simulink model "PubIfDecisionTOS_MDL"  (R2020b)
settings: configuration reference "DspaceConfig" (kept outside this file)
PostLoadFcn:
  | if any(exist('dsrtsu_mdlpostloadfcn', 'file') ~= 0), dsrtsu_mdlpostloadfcn('Execute', bdroot); end
InitFcn:
  | , if any(exist('dsmpb_private', 'file') ~= 0), dsmpb_private('dsmpb_mdlclblib', 'Init', bdroot); end,
undefined symbols (not defined in the file or in its folder): C_TOS_ACCEgoRAxletoFbumplength_m, C_TOS_ACCTargetFront_Flag, C_TOS_AEBJAPedObjDxThre_Val, C_TOS_AEBJAPedObjDyThre_Val, C_TOS_AEBJATargetSize_Val, C_TOS_AEBJAVehObjDxThre_Val, C_TOS_AEBJAVehObjDyThre_Val, C_TOS_AEBJuncPedTargetSize_Val, C_TOS_AEBLatObjDxThre_Val, C_TOS_AEBLatPedDyThre_Val, C_TOS_AEBLatTargetSize_Val, C_TOS_AEBLongTargetInEgoFront_Flag, C_TOS_axAbsGround_Parameter, C_TOS_CameraConfirmedFlag, C_TOS_CNsubjWidth, C_TOS_CurrentLaneCoreMinWidth_Val, C_TOS_CutInProb_Val_Zero, C_TOS_CutOutProb_Val_Zero, C_TOS_D2R_Val, C_TOS_DefaultValueObjectToCenterLine_dy, C_TOS_EgoCarWidth_Val, C_TOS_EgoDxRefPoint_m, C_TOS_EgoRAxletoFbumplength_m, C_TOS_HalfWidthVehicle_Con, C_TOS_HWA_CurrentLaneFlag, C_TOS_HWA_LeftLaneFlag, C_TOS_HWA_MovingDir_Vaild, C_TOS_HWA_MovState_Vaild, C_TOS_HWA_RightLaneFlag, C_TOS_LaneLineCourseErrorFront, C_TOS_LaneLineCourseErrorRear, C_TOS_MotorbikeDefaultWidth_m, C_TOS_NumberOfEffectiveTargets, C_TOS_Obj_Age_Val, C_TOS_Objdx_Constraint_Val, C_TOS_ObjectDefaultWidth_m, C_TOS_ObjInCurrentLane_Val, C_TOS_ObjInCurrentLaneValid, C_TOS_ObjInLeftLaneValid, C_TOS_ObjInRightLaneValid, C_TOS_ObjNotInCurrentLane_Val, C_TOS_ObjNotREElementType, C_TOS_ObjPredictDis_dy_ConstantVal_Zeros, C_TOS_ObjToCenterLine_ConstantVal_Zeros, C_TOS_OFMObjIDInvilad_Val, C_TOS_PIL_LatDisCons_Val_zero, C_TOS_PIL_ObjectCutInFlag_b, C_TOS_PIL_ObjectCutOutFlag_b, C_TOS_PIL_ObjLaneProb_al_Val, C_TOS_PP_ObjFusType_FC_Confirm_b, C_TOS_PP_ObjFusType_FC_FR_Confirm_b, C_TOS_PP_ObjFusType_FR_Confirm_b, C_TOS_RE_80BoolDefault_Val, C_TOS_RE_80Single181Default_Val, C_TOS_RE_80Single255Default_Val, C_TOS_RE_80Uint8Default_Val, C_TOS_RE_D2R, C_TOS_RE_D_180_Val, C_TOS_RE_InvalidObjectID_Val, C_TOS_RE_InvalidTargetChainDir_Val ... (+142)
libraries: simulink x1650, TOS_LIB x361, canfdmsglib x14
(part 31 of 69)

== system PubIfDecisionTOS_MDL/TOS_20201112/TOS_2012080320/TOS/LC_LCKie_ELK/TOS_HWA/RightLane/HWA_Object_PreConfirm/HWA_Object_PreConfirm ==
  PP_ObjFusType_FC_FR_Confirm : Inport  Partition=on  PartitionDimension=1  PartitionWidth=1  PartitionOffset=0
  PP_ObjFusType_FR_Confirm : Inport  Port=2  Partition=on  PartitionDimension=1  PartitionWidth=1  PartitionOffset=0
  PP_ObjFusType_FC_Confirm : Inport  Port=3  Partition=on  PartitionDimension=1  PartitionWidth=1  PartitionOffset=0
  Object_ID : Inport  Port=4  OutDataTypeStr=uint8  Partition=on  PartitionDimension=1  PartitionWidth=1  PartitionOffset=0
  Obj_MovingState : Inport  Port=5  Partition=on  PartitionDimension=1  PartitionWidth=1  PartitionOffset=0
  Obj_Dx : Inport  Port=6  Partition=on  PartitionDimension=1  PartitionWidth=1  PartitionOffset=0
  Object_ObstacleProb : Inport  Port=7  Partition=on  PartitionDimension=1  PartitionWidth=1  PartitionOffset=0
  Object_DY : Inport  Port=8  Partition=on  PartitionDimension=1  PartitionWidth=1  PartitionOffset=0
  Object_ObjType : Inport  Port=9  Partition=on  PartitionDimension=1  PartitionWidth=1  PartitionOffset=0
  Compare To Constant : simulink/Logic and Bit Operations/Compare To Constant  relop=~=  const=C_TOS_OFMObjIDInvilad_Val  OutDataTypeStr=boolean
      settings: AttributesFormatString=C_TOS_OFMObjIDInvilad_Val = 0
  Compare To Constant1 : simulink/Logic and Bit Operations/Compare To Constant  relop=>=  const=single(7)  OutDataTypeStr=boolean
      settings: AttributesFormatString=dx >= single(0)
  Compare To Constant2 : simulink/Logic and Bit Operations/Compare To Constant  relop=<  const=single(7)  OutDataTypeStr=boolean
      settings: AttributesFormatString=dx >= single(0)
  Default : Subsystem  TreatAsAtomicUnit=on
  For Each : ForEach  DisableCoverage=on
  HWA_Object_PreConfirm : Subsystem
  HWA_Object_PreConfirmDefault1 : Subsystem  TreatAsAtomicUnit=on
  If1 : If  NumInputs=2  IfExpression=u1 == 1  ElseIfExpressions=u2 == 1
  Logical Operator1 : Logic  AllPortsSameDT=off  OutDataTypeStr=boolean
  Logical Operator3 : Logic  AllPortsSameDT=off  OutDataTypeStr=boolean
  Merge{,1,3..5} (5 alike) : Merge  Inputs=3
  TOS_HWA_TargetPre_Confirm_Filt_Flag : Outport  ConcatenationDimension=1
  TOS_HWA_TargetPre_FusionTypeFlag_ObserVale : Outport  Port=2  ConcatenationDimension=1
  TOS_HWA_TargetPre_PassedbyTarget_ObserVale : Outport  Port=3  ConcatenationDimension=1
  TOS_HWA_TargetPre_ObjType_ObserVale : Outport  Port=4  ConcatenationDimension=1
  TOS_HWA_DyConfirm_ObserVale : Outport  Port=5  ConcatenationDimension=1
  wires:
  PP_ObjFusType_FC_FR_Confirm/1 -> HWA_Object_PreConfirm/2(PP_ObjFusType_FC_FR_Confirm)
  PP_ObjFusType_FR_Confirm/1 -> HWA_Object_PreConfirm/3(PP_ObjFusType_FR_Confirm)
  Compare To Constant/1 -> Logical Operator1/1, Logical Operator3/1
  Object_ID/1 -> [Object_ID], Compare To Constant/1
  If1/3 -> Default/Action
  If1/1 -> HWA_Object_PreConfirm/Action
  PP_ObjFusType_FC_Confirm/1 -> HWA_Object_PreConfirm/4(PP_ObjFusType_FC_Confirm)
  Obj_MovingState/1 -> HWA_Object_PreConfirm/5(Obj_MovingState)
  Obj_Dx/1 -> HWA_Object_PreConfirm/6(Obj_Dx)
  Object_ObstacleProb/1 -> HWA_Object_PreConfirm/7(Object_ObstacleProb)
  Object_DY/1 -> HWA_Object_PreConfirm/8(Object_DY)
  [Object_ID] -> HWA_Object_PreConfirm/1(Object_ID)
  Object_ObjType/1 -> HWA_Object_PreConfirm/9(Object_ObjType)
  HWA_Object_PreConfirm/1(TOS_HWA_TargetPre_Confirm_Filt_Flag) -> Merge/2
  HWA_Object_PreConfirm/2(TOS_HWA_TargetPre_FusionTypeFlag_ObserVale) -> Merge5/2
  HWA_Object_PreConfirm/3(TOS_HWA_TargetPre_PassedbyTarget_Flag_ObserVale) -> Merge1/2
  HWA_Object_PreConfirm/4(TOS_HWA_TargetPre_ObjType_ObserVale) -> Merge3/2
  HWA_Object_PreConfirm/5(TOS_HWA_DyConfirm_ObserVale) -> Merge4/2
  Merge/1 -> TOS_HWA_TargetPre_Confirm_Filt_Flag/1
  Merge5/1 -> TOS_HWA_TargetPre_FusionTypeFlag_ObserVale/1
  Merge1/1 -> TOS_HWA_TargetPre_PassedbyTarget_ObserVale/1
  Merge3/1 -> TOS_HWA_TargetPre_ObjType_ObserVale/1
  Merge4/1 -> TOS_HWA_DyConfirm_ObserVale/1
  [Obj_Dx] -> Compare To Constant1/1, Compare To Constant2/1
  Compare To Constant1/1 -> Logical Operator3/2
  Compare To Constant2/1 -> Logical Operator1/2
  Logical Operator3/1 -> If1/1
  Logical Operator1/1 -> If1/2
  If1/2 -> HWA_Object_PreConfirmDefault1/Action
  HWA_Object_PreConfirmDefault1/1(TOS_HWA_TargetPre_Confirm_Filt_Flag) -> Merge/1
  HWA_Object_PreConfirmDefault1/2(TOS_HWA_TargetPre_FusionTypeFlag_ObserVale) -> Merge5/1
  HWA_Object_PreConfirmDefault1/3(TOS_HWA_TargetPre_PassedbyTarget_Flag_ObserVale) -> Merge1/1
  HWA_Object_PreConfirmDefault1/4(TOS_HWA_TargetPre_ObjType_ObserVale) -> Merge3/1
  HWA_Object_PreConfirmDefault1/5(TOS_HWA_DyConfirm_ObserVale) -> Merge4/1
  Default/5(TOS_HWA_DyConfirm_ObserVale) -> Merge4/3
  Default/4(TOS_HWA_TargetPre_ObjType_ObserVale) -> Merge3/3
  Default/3(TOS_HWA_TargetPre_PassedbyTarget_Flag_ObserVale) -> Merge1/3
  Default/2(TOS_HWA_TargetPre_FusionTypeFlag_ObserVale) -> Merge5/3
  Default/1(TOS_HWA_TargetPre_Confirm_Filt_Flag) -> Merge/3

== system PubIfDecisionTOS_MDL/TOS_20201112/TOS_2012080320/TOS/LC_LCKie_ELK/TOS_HWA/RightLane/TOS_HWA_RightLane/TOS_HWA_RightLane ==
  HWA_RightLane_ObjIndex : Inport  Partition=on  PartitionDimension=1  PartitionWidth=1  PartitionOffset=0
  PP_ObjMovingDirSignalProcessing : Inport  Port=2
  Object_VX : Inport  Port=3
  Object_VY : Inport  Port=4
  Object_Type : Inport  Port=5
  Object_MovingState : Inport  Port=6
  TOS_TLJ_RightLaneConfirm_Flag : Inport  Port=7
  Object_DX : Inport  Port=8
  Object_DY : Inport  Port=9
  Object_Fus_Type : Inport  Port=10
  Object_HeadingAngle : Inport  Port=11
  PP_ObjFusType_FC_FR_Confirm : Inport  Port=12
  PP_ObjFusType_FR_Confirm : Inport  Port=13
  PP_ObjFusType_FC_Confirm : Inport  Port=14
  VIE_EgoVelocity : Inport  Port=15
  Compare To Constant : simulink/Logic and Bit Operations/Compare To Constant  relop===  const=C_TOS_OFMObjIDInvilad_Val  OutDataTypeStr=boolean
      settings: AttributesFormatString=C_TOS_OFMObjIDInvilad_Val = 0
  Constant : Constant  Value=0  OutDataTypeStr=uint8
  Constant1 : Constant  Value=0  OutDataTypeStr=uint8
  Constant2 : Constant  Value=0  OutDataTypeStr=uint8
  Constant4 : Constant  Value=C_TOS_ObjInRightLaneValid  OutDataTypeStr=uint8
      settings: AttributesFormatString=C_TOS_ObjInRightLaneValid = 3
  For Each : ForEach  DisableCoverage=on
  If : If  IfExpression=u1 ~= 0
  Merge{1..11} (11 alike) : Merge
  Switch : Switch  Criteria=u2 ~= 0
  Switch1 : Switch  Criteria=u2 ~= 0
  Switch2 : Switch  Criteria=u2 ~= 0
  TOS_HWA : Subsystem
  TOS_HWA_Default : Subsystem  TreatAsAtomicUnit=on
  TOS_HWA_TargetInRightLane_b : Outport  ConcatenationDimension=1
  TOS_HWA_RightFront_TargConfirm_b : Outport  Port=2  ConcatenationDimension=1
  TOS_HWA_RightRear_TargConfirm_b : Outport  Port=3  ConcatenationDimension=1
  TOS_HWA_RightFront_FusType_ObserVale : Outport  Port=4  ConcatenationDimension=1
  TOS_HWA_InRightLane_Front_Flag_ObserVale : Outport  Port=5  ConcatenationDimension=1
  TOS_HWA_RightFront_TargMovDir_ObserVale : Outport  Port=6  ConcatenationDimension=1
  TOS_HWA_RightRear_MovState_ObserVale : Outport  Port=7  ConcatenationDimension=1
  TOS_HWA_RightRear_FusionType_ObserVale : Outport  Port=8  ConcatenationDimension=1
  TOS_HWA_InRightLane_Rear_Flag_ObserVale : Outport  Port=9  ConcatenationDimension=1
  TOS_HWA_RightRear_TargetMovingDir_ObserVale : Outport  Port=10  ConcatenationDimension=1
  TOS_HWA_RightRear_DyConfirm_ObserVale : Outport  Port=11  ConcatenationDimension=1
  wires:
  If/1 -> TOS_HWA_Default/Action
  Compare To Constant/1 -> If/1
  If/2 -> TOS_HWA/Action
  PP_ObjMovingDirSignalProcessing/1 -> TOS_HWA/2(PP_ObjMovingDirSignalProcessing)
  Object_VX/1 -> TOS_HWA/3(Object_VX)
  Object_VY/1 -> TOS_HWA/4(Object_VY)
  Object_Type/1 -> TOS_HWA/5(Object_Type)
  Object_MovingState/1 -> TOS_HWA/6(object_MovingState)
  TOS_TLJ_RightLaneConfirm_Flag/1 -> TOS_HWA/7(TOS_TLJ_RightLaneConfirm_Flag)
  Object_DX/1 -> TOS_HWA/8(Object_DX)  "Object_DX"
  Object_Fus_Type/1 -> TOS_HWA/10(Object_Fus_Type)
  Object_HeadingAngle/1 -> TOS_HWA/11(Object_HeadingAngle)  "Object_HeadingAngle"
  HWA_RightLane_ObjIndex/1 -> [HWA_RightLane_ObjIndex], Compare To Constant/1
  [HWA_RightLane_ObjIndex] -> Switch/1
  Constant/1 -> Switch/3
  Switch/1 -> TOS_HWA_RightFront_TargConfirm_b/1
  Switch1/1 -> TOS_HWA_RightRear_TargConfirm_b/1
  Constant1/1 -> Switch1/3
  [HWA_RightLane_ObjIndex] -> Switch1/1
  [HWA_RightLane_ObjIndex] -> TOS_HWA/1(HWA_RightLane_ObjIndex)
  Constant4/1 -> Switch2/1
  Constant2/1 -> Switch2/3
  Switch2/1 -> TOS_HWA_TargetInRightLane_b/1
  PP_ObjFusType_FC_Confirm/1 -> TOS_HWA/14(PP_ObjFusType_FC_Confirm)
  PP_ObjFusType_FC_FR_Confirm/1 -> TOS_HWA/12(PP_ObjFusType_FC_FR_Confirm)
  PP_ObjFusType_FR_Confirm/1 -> TOS_HWA/13(PP_ObjFusType_FR_Confirm)
  VIE_EgoVelocity/1 -> TOS_HWA/15(VIE_EgoVelocity)
  TOS_HWA/11(TOS_HWA_RightRear_DyConfirm_ObserVale) -> Merge11/2
  TOS_HWA/1(TOS_HWA_TargetInRightLane_b) -> Merge3/2
  TOS_HWA/2(TOS_HWA_RightFront_TargConfirm_b) -> Merge4/2
  TOS_HWA/3(TOS_HWA_RightRear_TargConfirm_b) -> Merge5/2
  TOS_HWA/4(TOS_HWA_RightFront_FusType_ObserVale) -> Merge1/2
  TOS_HWA/5(TOS_HWA_InRightLane_Front_Flag_ObserVale) -> Merge2/2
  TOS_HWA/6(TOS_HWA_RightFront_TargMovDir_ObserVale) -> Merge6/2
  TOS_HWA/7(TOS_HWA_RightRear_MovState_ObserVale) -> Merge7/2
  TOS_HWA/8(TOS_HWA_RightRear_FusionType_ObserVale) -> Merge8/2
  TOS_HWA/9(TOS_HWA_InRightLane_Rear_Flag_ObserVale) -> Merge9/2
  TOS_HWA/10(TOS_HWA_RightRear_TargetMovingDir_ObserVale) -> Merge10/2
  TOS_HWA_Default/1(TOS_HWA_TargetInRightLane_b) -> Merge3/1
  Merge4/1 -> Switch/2
  Merge5/1 -> Switch1/2
  TOS_HWA_Default/2(TOS_HWA_RightFront_TargConfirm_b) -> Merge4/1
  TOS_HWA_Default/3(TOS_HWA_RightRear_TargConfirm_b) -> Merge5/1
  Merge3/1 -> Switch2/2
  Merge1/1 -> TOS_HWA_RightFront_FusType_ObserVale/1
  Merge11/1 -> TOS_HWA_RightRear_DyConfirm_ObserVale/1
  Merge2/1 -> TOS_HWA_InRightLane_Front_Flag_ObserVale/1
  Merge6/1 -> TOS_HWA_RightFront_TargMovDir_ObserVale/1
  Merge7/1 -> TOS_HWA_RightRear_MovState_ObserVale/1
  Merge8/1 -> TOS_HWA_RightRear_FusionType_ObserVale/1
  Merge9/1 -> TOS_HWA_InRightLane_Rear_Flag_ObserVale/1
  Merge10/1 -> TOS_HWA_RightRear_TargetMovingDir_ObserVale/1
  TOS_HWA_Default/4(TOS_HWA_RightFront_FusType_ObserVale) -> Merge1/1
  TOS_HWA_Default/5(TOS_HWA_InRightLane_Front_Flag_ObserVale) -> Merge2/1
  TOS_HWA_Default/6(TOS_HWA_RightFront_TargMovDir_ObserVale) -> Merge6/1
  TOS_HWA_Default/7(TOS_HWA_RightRear_MovState_ObserVale) -> Merge7/1
  TOS_HWA_Default/8(TOS_HWA_RightRear_FusionType_ObserVale) -> Merge8/1
  TOS_HWA_Default/9(TOS_HWA_InRightLane_Rear_Flag_ObserVale) -> Merge9/1
  TOS_HWA_Default/10(TOS_HWA_RightRear_TargetMovingDir_ObserVale) -> Merge10/1
  TOS_HWA_Default/11(TOS_HWA_RightRear_DyConfirm_ObserVale) -> Merge11/1
  Object_DY/1 -> TOS_HWA/9(Object_DY)  "Object_DY"

== system PubIfDecisionTOS_MDL/TOS_20201112/TOS_2012080320/TOS/P0_Trajectory_V1.0/CordinatConvert/CordinatConvert/CordinatConvert/TrackRecord_CordinatConvert ==
  note: 清除后方 -20m以后目标（不清除，历史点一直存在对下一次拟合有影响）
  note: 默认数组，无目标时，不坐标转换
  EgoVeh_OffsetX : Inport
  EgoVeh_OffsetY : Inport  Port=2
  EgoVeh_OffsetAngle : Inport  Port=3
  P0_dx_TrackRecord_K1 : Inport  Port=4  Partition=on  PartitionDimension=1  PartitionWidth=1  PartitionOffset=0
  P0_dy_TrackRecord_K1 : Inport  Port=5  Partition=on  PartitionDimension=1  PartitionWidth=1  PartitionOffset=0
  P0_Counter_TrackRecord : Inport  Port=6  Partition=on  PartitionDimension=1  PartitionWidth=1  PartitionOffset=0
  P0_ID_TrackRecord_K1 : Inport  Port=7  Partition=on  PartitionDimension=1  PartitionWidth=1  PartitionOffset=0
  Bus Creator : BusCreator  Inputs=7
  Bus Selector : BusSelector  OutputSignals=P0_dx_TrackRecord_K1,P0_dy_TrackRecord_K1,P0_Counter_TrackRecord
  Bus Selector1 : BusSelector  OutputSignals=EgoVeh_OffsetX,EgoVeh_OffsetY,EgoVeh_OffsetAngle,P0_dx_TrackRecord_K1,P0_dy_TrackRecord_K1,P0_Counter_TrackRecord,P0_ID_TrackRecord_K1
  Bus Selector2 : BusSelector  OutputSignals=P0_dx_TrackRecord_K1
  Compare To Constant : simulink/Logic and Bit Operations/Compare To Constant  relop===  const=single(0)  OutDataTypeStr=boolean
      settings: AttributesFormatString=Invilad_Val = single(0)
  Compare To Constant1 : simulink/Logic and Bit Operations/Compare To Constant  relop===  const=single(0)  OutDataTypeStr=boolean
      settings: AttributesFormatString=Invilad_Val = single(0)
  Compare To Constant2 : simulink/Logic and Bit Operations/Compare To Constant  relop===  const=uint32(0)  OutDataTypeStr=boolean
      settings: AttributesFormatString=Invilad_Val = uint32(0)
  Compare To Constant3 : simulink/Logic and Bit Operations/Compare To Constant  relop=<=  const=single(-20)  OutDataTypeStr=boolean
      settings: AttributesFormatString=single(-20)
  CordinatConvertDefault : Subsystem  TreatAsAtomicUnit=on
  For Each : ForEach  DisableCoverage=on
  If : If  IfExpression=u1 == 1
  Logical Operator1 : Logic  Inputs=3  AllPortsSameDT=off  OutDataTypeStr=boolean
  Logical Operator2 : Logic  Operator=OR  AllPortsSameDT=off  OutDataTypeStr=boolean
  Merge{1..4} (4 alike) : Merge
  TrackRecord_CordinatConvert : Subsystem
  P0_dx_TrackRecord_CordinatConvert_K1 : Outport  ConcatenationDimension=1
  P0_dy_TrackRecord_CordinatConvert_K1 : Outport  Port=2  ConcatenationDimension=1
  P0_Counter_TrackRecord_CordinatConvert_K1 : Outport  Port=3  ConcatenationDimension=1
  P0_ID_TrackRecord_CordinatConvert_K1 : Outport  Port=4  ConcatenationDimension=1
  wires:
  Merge3/1 -> P0_Counter_TrackRecord_CordinatConvert_K1/1
  Merge1/1 -> P0_dy_TrackRecord_CordinatConvert_K1/1
  Merge2/1 -> P0_dx_TrackRecord_CordinatConvert_K1/1
  CordinatConvertDefault/3(P0_Counter_TrackRecord_CordinatConvert_K1) -> Merge3/1
  CordinatConvertDefault/2(P0_dy_TrackRecord_CordinatConvert_K1) -> Merge1/1
  CordinatConvertDefault/1(P0_dx_TrackRecord_CordinatConvert_K1) -> Merge2/1
  TrackRecord_CordinatConvert/3(P0_Counter_TrackRecord_CordinatConvert_K1) -> Merge3/2
  TrackRecord_CordinatConvert/2(P0_dy_TrackRecord_CordinatConvert_K1) -> Merge1/2
  TrackRecord_CordinatConvert/1(P0_dx_TrackRecord_CordinatConvert_K1) -> Merge2/2
  Bus Selector1/6 -> TrackRecord_CordinatConvert/6(P0_Counter_TrackRecord)  "<P0_Counter_TrackRecord>"
  Bus Selector1/5 -> TrackRecord_CordinatConvert/5(P0_dy_TrackRecord_K1)  "<P0_dy_TrackRecord_K1>"
  Bus Selector1/4 -> TrackRecord_CordinatConvert/4(P0_dx_TrackRecord_K1)  "<P0_dx_TrackRecord_K1>"
  Bus Selector1/3 -> TrackRecord_CordinatConvert/3(EgoVeh_OffsetAngle)  "<EgoVeh_OffsetAngle>"
  Bus Selector1/2 -> TrackRecord_CordinatConvert/2(EgoVeh_OffsetY)  "<EgoVeh_OffsetY>"
  Bus Selector1/1 -> TrackRecord_CordinatConvert/1(EgoVeh_OffsetX)  "<EgoVeh_OffsetX>"
  [TrackRecord_CordinatConvert] -> Bus Selector1/1
  If/2 -> TrackRecord_CordinatConvert/Action
  If/1 -> CordinatConvertDefault/Action
  Logical Operator2/1 -> If/1
  Compare To Constant2/1 -> Logical Operator1/3
  Compare To Constant1/1 -> Logical Operator1/2
  Compare To Constant/1 -> Logical Operator1/1
  Bus Selector/3 -> Compare To Constant2/1  "<P0_Counter_TrackRecord>"
  Bus Selector/2 -> Compare To Constant1/1  "<P0_dy_TrackRecord_K1>"
  Bus Selector/1 -> Compare To Constant/1  "<P0_dx_TrackRecord_K1>"
  Bus Creator/1 -> Bus Selector2/1, Bus Selector/1, [TrackRecord_CordinatConvert]
  EgoVeh_OffsetY/1 -> Bus Creator/2  "EgoVeh_OffsetY"
  EgoVeh_OffsetAngle/1 -> Bus Creator/3  "EgoVeh_OffsetAngle"
  P0_Counter_TrackRecord/1 -> Bus Creator/6  "P0_Counter_TrackRecord"
  P0_dy_TrackRecord_K1/1 -> Bus Creator/5  "P0_dy_TrackRecord_K1"
  EgoVeh_OffsetX/1 -> Bus Creator/1  "EgoVeh_OffsetX"
  P0_dx_TrackRecord_K1/1 -> Bus Creator/4  "P0_dx_TrackRecord_K1"
  P0_ID_TrackRecord_K1/1 -> Bus Creator/7  "P0_ID_TrackRecord_K1"
  Bus Selector1/7 -> TrackRecord_CordinatConvert/7(P0_ID_TrackRecord_K1)  "<P0_ID_TrackRecord_K1>"
  Merge4/1 -> P0_ID_TrackRecord_CordinatConvert_K1/1
  TrackRecord_CordinatConvert/4(P0_ID_TrackRecord_CordinatConvert_K2) -> Merge4/2
  CordinatConvertDefault/4(P0_ID_TrackRecord_CordinatConvert_K1) -> Merge4/1
  Bus Selector2/1 -> Compare To Constant3/1  "<P0_dx_TrackRecord_K1>"
  Compare To Constant3/1 -> Logical Operator2/2
  Logical Operator1/1 -> Logical Operator2/1

== system PubIfDecisionTOS_MDL/TOS_20201112/TOS_2012080320/TOS/P0_Trajectory_V1.0/CordinatConvert/CordinatConvert1/CordinatConvert/TrackRecord_CordinatConvert ==
  note: 默认数组，无目标时，不坐标转换
  note: 清除后方 -20m以后目标（不清除，历史点一直存在对下一次拟合有影响）
  EgoVeh_OffsetX : Inport
  EgoVeh_OffsetY : Inport  Port=2
  EgoVeh_OffsetAngle : Inport  Port=3
  P0_dx_TrackRecord_K1 : Inport  Port=4  Partition=on  PartitionDimension=1  PartitionWidth=1  PartitionOffset=0
  P0_dy_TrackRecord_K1 : Inport  Port=5  Partition=on  PartitionDimension=1  PartitionWidth=1  PartitionOffset=0
  P0_Counter_TrackRecord : Inport  Port=6  Partition=on  PartitionDimension=1  PartitionWidth=1  PartitionOffset=0
  P0_ID_TrackRecord_K1 : Inport  Port=7  Partition=on  PartitionDimension=1  PartitionWidth=1  PartitionOffset=0
  Bus Creator : BusCreator  Inputs=7
  Bus Selector : BusSelector  OutputSignals=P0_dx_TrackRecord_K1,P0_dy_TrackRecord_K1,P0_Counter_TrackRecord
  Bus Selector1 : BusSelector  OutputSignals=EgoVeh_OffsetX,EgoVeh_OffsetY,EgoVeh_OffsetAngle,P0_dx_TrackRecord_K1,P0_dy_TrackRecord_K1,P0_Counter_TrackRecord,P0_ID_TrackRecord_K1
  Bus Selector2 : BusSelector  OutputSignals=P0_dx_TrackRecord_K1
  Compare To Constant : simulink/Logic and Bit Operations/Compare To Constant  relop===  const=single(0)  OutDataTypeStr=boolean
      settings: AttributesFormatString=Invilad_Val = single(0)
  Compare To Constant1 : simulink/Logic and Bit Operations/Compare To Constant  relop===  const=single(0)  OutDataTypeStr=boolean
      settings: AttributesFormatString=Invilad_Val = single(0)
  Compare To Constant2 : simulink/Logic and Bit Operations/Compare To Constant  relop===  const=uint32(0)  OutDataTypeStr=boolean
      settings: AttributesFormatString=Invilad_Val = uint32(0)
  Compare To Constant3 : simulink/Logic and Bit Operations/Compare To Constant  relop=<=  const=single(-20)  OutDataTypeStr=boolean
      settings: AttributesFormatString=single(-20)
  CordinatConvertDefault : Subsystem  TreatAsAtomicUnit=on
  For Each : ForEach  DisableCoverage=on
  If : If  IfExpression=u1 == 1
  Logical Operator1 : Logic  Inputs=3  AllPortsSameDT=off  OutDataTypeStr=boolean
  Logical Operator2 : Logic  Operator=OR  AllPortsSameDT=off  OutDataTypeStr=boolean
  Merge{1..4} (4 alike) : Merge
  TrackRecord_CordinatConvert : Subsystem
  P0_dx_TrackRecord_CordinatConvert_K1 : Outport  ConcatenationDimension=1
  P0_dy_TrackRecord_CordinatConvert_K1 : Outport  Port=2  ConcatenationDimension=1
  P0_Counter_TrackRecord_CordinatConvert_K1 : Outport  Port=3  ConcatenationDimension=1
  P0_ID_TrackRecord_CordinatConvert_K1 : Outport  Port=4  ConcatenationDimension=1
  wires:
  Logical Operator1/1 -> Logical Operator2/1
  Compare To Constant3/1 -> Logical Operator2/2
  Bus Selector2/1 -> Compare To Constant3/1  "<P0_dx_TrackRecord_K1>"
  CordinatConvertDefault/4(P0_ID_TrackRecord_CordinatConvert_K1) -> Merge4/1
  TrackRecord_CordinatConvert/4(P0_ID_TrackRecord_CordinatConvert_K2) -> Merge4/2
  Merge4/1 -> P0_ID_TrackRecord_CordinatConvert_K1/1
  Bus Selector1/7 -> TrackRecord_CordinatConvert/7(P0_ID_TrackRecord_K1)  "<P0_ID_TrackRecord_K1>"
  P0_ID_TrackRecord_K1/1 -> Bus Creator/7  "P0_ID_TrackRecord_K1"
  P0_dx_TrackRecord_K1/1 -> Bus Creator/4  "P0_dx_TrackRecord_K1"
  EgoVeh_OffsetX/1 -> Bus Creator/1  "EgoVeh_OffsetX"
  P0_dy_TrackRecord_K1/1 -> Bus Creator/5  "P0_dy_TrackRecord_K1"
  P0_Counter_TrackRecord/1 -> Bus Creator/6  "P0_Counter_TrackRecord"
  EgoVeh_OffsetAngle/1 -> Bus Creator/3  "EgoVeh_OffsetAngle"
  EgoVeh_OffsetY/1 -> Bus Creator/2  "EgoVeh_OffsetY"
  Bus Creator/1 -> [TrackRecord_CordinatConvert], Bus Selector/1, Bus Selector2/1
  Bus Selector/1 -> Compare To Constant/1  "<P0_dx_TrackRecord_K1>"
  Bus Selector/2 -> Compare To Constant1/1  "<P0_dy_TrackRecord_K1>"
  Bus Selector/3 -> Compare To Constant2/1  "<P0_Counter_TrackRecord>"
  Compare To Constant/1 -> Logical Operator1/1
  Compare To Constant1/1 -> Logical Operator1/2
  Compare To Constant2/1 -> Logical Operator1/3
  Logical Operator2/1 -> If/1
  If/1 -> CordinatConvertDefault/Action
  If/2 -> TrackRecord_CordinatConvert/Action
  [TrackRecord_CordinatConvert] -> Bus Selector1/1
  Bus Selector1/1 -> TrackRecord_CordinatConvert/1(EgoVeh_OffsetX)  "<EgoVeh_OffsetX>"
  Bus Selector1/2 -> TrackRecord_CordinatConvert/2(EgoVeh_OffsetY)  "<EgoVeh_OffsetY>"
  Bus Selector1/3 -> TrackRecord_CordinatConvert/3(EgoVeh_OffsetAngle)  "<EgoVeh_OffsetAngle>"
  Bus Selector1/4 -> TrackRecord_CordinatConvert/4(P0_dx_TrackRecord_K1)  "<P0_dx_TrackRecord_K1>"
  Bus Selector1/5 -> TrackRecord_CordinatConvert/5(P0_dy_TrackRecord_K1)  "<P0_dy_TrackRecord_K1>"
  Bus Selector1/6 -> TrackRecord_CordinatConvert/6(P0_Counter_TrackRecord)  "<P0_Counter_TrackRecord>"
  TrackRecord_CordinatConvert/1(P0_dx_TrackRecord_CordinatConvert_K1) -> Merge2/2
  TrackRecord_CordinatConvert/2(P0_dy_TrackRecord_CordinatConvert_K1) -> Merge1/2
  TrackRecord_CordinatConvert/3(P0_Counter_TrackRecord_CordinatConvert_K1) -> Merge3/2
  CordinatConvertDefault/1(P0_dx_TrackRecord_CordinatConvert_K1) -> Merge2/1
  CordinatConvertDefault/2(P0_dy_TrackRecord_CordinatConvert_K1) -> Merge1/1
  CordinatConvertDefault/3(P0_Counter_TrackRecord_CordinatConvert_K1) -> Merge3/1
  Merge2/1 -> P0_dx_TrackRecord_CordinatConvert_K1/1
  Merge1/1 -> P0_dy_TrackRecord_CordinatConvert_K1/1
  Merge3/1 -> P0_Counter_TrackRecord_CordinatConvert_K1/1

== system PubIfDecisionTOS_MDL/TOS_20201112/TOS_2012080320/TOS/P0_Trajectory_V1.0/TrackRecord/Subsystem1/P0_Position_Num/EndPosition ==
  P0_dx_TrackRecord_CordinatConvert_K1 : Inport
  P0_dy_TrackRecord_CordinatConvert_K1 : Inport  Port=2
  P0_ObjVaild_TrackRecord_CordinatConvert_K1 : Inport  Port=3
  P0_Trajectory_TrackRecord_Num : Inport  Port=4
  Abs : Abs
  Abs1 : Abs
  Abs2 : Abs
  Add : Sum  OutDataTypeStr=int32
  Compare To Constant1 : simulink/Logic and Bit Operations/Compare To Constant  relop=~=  const=single(0)  OutDataTypeStr=boolean
      settings: AttributesFormatString=single(0)
  Compare To Constant10 : simulink/Logic and Bit Operations/Compare To Constant  relop===  const=uint32(0)  OutDataTypeStr=boolean
      settings: AttributesFormatString=uint32(0)
  Compare To Constant2 : simulink/Logic and Bit Operations/Compare To Constant  relop=~=  const=uint32(0)  OutDataTypeStr=boolean
      settings: AttributesFormatString=uint32(0)
  Compare To Constant5 : simulink/Logic and Bit Operations/Compare To Constant  relop=~=  const=single(0)  OutDataTypeStr=boolean
      settings: AttributesFormatString=single(0)
  Constant : Constant  OutDataTypeStr=int32
  Data Type Conversion : DataTypeConversion  OutDataTypeStr=uint32
  Index Vector{,1..5} (6 alike) : MultiPortSwitch  Inputs=1
  Logical Operator2 : Logic  Inputs=4  AllPortsSameDT=off  OutDataTypeStr=boolean
  P0_dx_TrackRecord_CordinatConvert_K2 : InportShadow
  P0_dy_TrackRecord_CordinatConvert_K2 : InportShadow  Port=2
  Saturation : Saturate  UpperLimit=int32(P_TOS_P0_Trajectory_TrackRecord_Num)  LowerLimit=int32(1)
  Saturation1 : Saturate  UpperLimit=int32(P_TOS_P0_Trajectory_TrackRecord_Num)  LowerLimit=int32(1)
  Switch : Switch  Criteria=u2 > Threshold
  Unit Delay13 : UnitDelay  InitialCondition=uint32(1)  SampleTime=-1  HasFrameUpgradeWarning=on
      settings: AttributesFormatString=%<InitialCondition>
  P0_EndPosition_Num : Outport
  P0_EndPosition_dx : Outport  Port=2
  P0_EndPosition_dy : Outport  Port=3
  wires:
  Index Vector4/1 -> P0_EndPosition_dx/1
  P0_dx_TrackRecord_CordinatConvert_K2/1 -> Index Vector4/2
  Saturation1/1 -> Switch/1
  Switch/1 -> Unit Delay13/1, Index Vector5/1, Index Vector4/1, P0_EndPosition_Num/1
  Unit Delay13/1 -> Switch/3
  P0_Trajectory_TrackRecord_Num/1 -> Data Type Conversion/1, Index Vector1/1, Index Vector2/1, Add/2, Index Vector/1
  Data Type Conversion/1 -> Saturation1/1
  Logical Operator2/1 -> Switch/2
  Compare To Constant10/1 -> Logical Operator2/4
  Index Vector3/1 -> Compare To Constant10/1
  Compare To Constant2/1 -> Logical Operator2/3
  Compare To Constant1/1 -> Logical Operator2/2
  Compare To Constant5/1 -> Logical Operator2/1
  Saturation/1 -> Index Vector3/1
  Add/1 -> Saturation/1
  Constant/1 -> Add/1
  Abs2/1 -> Compare To Constant2/1
  Abs/1 -> Compare To Constant1/1
  Abs1/1 -> Compare To Constant5/1
  Index Vector/1 -> Abs1/1
  Index Vector2/1 -> Abs2/1
  P0_ObjVaild_TrackRecord_CordinatConvert_K1/1 -> Index Vector2/2, Index Vector3/2
  P0_dy_TrackRecord_CordinatConvert_K1/1 -> Index Vector/2
  P0_dx_TrackRecord_CordinatConvert_K1/1 -> Index Vector1/2
  Index Vector1/1 -> Abs/1
  P0_dy_TrackRecord_CordinatConvert_K2/1 -> Index Vector5/2
  Index Vector5/1 -> P0_EndPosition_dy/1

== system PubIfDecisionTOS_MDL/TOS_20201112/TOS_2012080320/TOS/P0_Trajectory_V1.0/TrackRecord/Subsystem1/P0_Position_Num/StartPosition ==
  P0_dx_TrackRecord_CordinatConvert_K1 : Inport
  P0_dy_TrackRecord_CordinatConvert_K1 : Inport  Port=2
  P0_ObjVaild_TrackRecord_CordinatConvert_K1 : Inport  Port=3
  P0_Trajectory_TrackRecord_Num : Inport  Port=4
  Abs : Abs
  Abs1 : Abs
  Abs2 : Abs
  Add : Sum  OutDataTypeStr=int32
  Add1 : Sum
  Compare To Constant1 : simulink/Logic and Bit Operations/Compare To Constant  relop===  const=single(0)  OutDataTypeStr=boolean
      settings: AttributesFormatString=single(0)
  Compare To Constant10 : simulink/Logic and Bit Operations/Compare To Constant  relop=~=  const=uint32(0)  OutDataTypeStr=boolean
      settings: AttributesFormatString=uint32(0)
  Compare To Constant2 : simulink/Logic and Bit Operations/Compare To Constant  relop===  const=uint32(0)  OutDataTypeStr=boolean
      settings: AttributesFormatString=uint32(0)
  Compare To Constant5 : simulink/Logic and Bit Operations/Compare To Constant  relop===  const=single(0)  OutDataTypeStr=boolean
      settings: AttributesFormatString=single(0)
  Constant : Constant  OutDataTypeStr=int32
  Constant1 : Constant  OutDataTypeStr=uint32
  Data Type Conversion : DataTypeConversion  OutDataTypeStr=uint32
  Index Vector{,1..4} (5 alike) : MultiPortSwitch  Inputs=1
  Logical Operator2 : Logic  Inputs=4  AllPortsSameDT=off  OutDataTypeStr=boolean
  P0_dx_TrackRecord_CordinatConvert_K1_1 : InportShadow
  Saturation : Saturate  UpperLimit=int32(P_TOS_P0_Trajectory_TrackRecord_Num)  LowerLimit=int32(1)
  Saturation1 : Saturate  UpperLimit=int32(P_TOS_P0_Trajectory_TrackRecord_Num)  LowerLimit=int32(1)
  Switch : Switch  Criteria=u2 > Threshold
  Unit Delay13 : UnitDelay  InitialCondition=uint32(1)  SampleTime=-1  HasFrameUpgradeWarning=on
      settings: AttributesFormatString=%<InitialCondition>
  P0_StartPosition_Num : Outport
  P0_StartPosition_Dis : Outport  Port=2
  wires:
  P0_ObjVaild_TrackRecord_CordinatConvert_K1/1 -> Index Vector3/2, Index Vector2/2
  Index Vector1/1 -> Abs/1
  P0_Trajectory_TrackRecord_Num/1 -> Index Vector/1, Add/2, Index Vector2/1, Index Vector1/1, Data Type Conversion/1
  Abs2/1 -> Compare To Constant2/1
  Abs/1 -> Compare To Constant1/1
  P0_dy_TrackRecord_CordinatConvert_K1/1 -> Index Vector/2
  Index Vector4/1 -> P0_StartPosition_Dis/1
  Index Vector/1 -> Abs1/1
  Constant1/1 -> Add1/1
  Abs1/1 -> Compare To Constant5/1
  Compare To Constant5/1 -> Logical Operator2/1
  Saturation/1 -> Index Vector3/1
  Constant/1 -> Add/1
  Unit Delay13/1 -> Switch/3
  P0_dx_TrackRecord_CordinatConvert_K1_1/1 -> Index Vector4/2
  Saturation1/1 -> Switch/1
  Add/1 -> Saturation/1
  Index Vector2/1 -> Abs2/1
  Index Vector3/1 -> Compare To Constant10/1
  Logical Operator2/1 -> Switch/2
  Add1/1 -> Saturation1/1
  Compare To Constant1/1 -> Logical Operator2/2
  Switch/1 -> P0_StartPosition_Num/1, Index Vector4/1, Unit Delay13/1
  Compare To Constant10/1 -> Logical Operator2/4
  P0_dx_TrackRecord_CordinatConvert_K1/1 -> Index Vector1/2
  Compare To Constant2/1 -> Logical Operator2/3
  Data Type Conversion/1 -> Add1/2

== system PubIfDecisionTOS_MDL/TOS_20201112/TOS_2012080320/TOS/P0_Trajectory_V1.0/TrgValidConfirm/TrgValidConfirm/TrgValidConfirm/TrgValidConfirm ==
  TrgValidConfirm_inf : Inport
  Action Port : ActionPort  ActionPortLabel=if(u1 == 1)
  Add : Sum
  Bus Selector1 : BusSelector  OutputSignals=P0_Counter_K1
  Bus Selector2 : BusSelector  OutputSignals=IDP0,dxP0,ObjDYP0
  Constant2 : Constant  OutDataTypeStr=uint32
  P0_ID : Outport
  P0_Counter : Outport  Port=2
  P0_dx : Outport  Port=3
  P0_dy : Outport  Port=4
  wires:
  Bus Selector1/1 -> Add/1  "<P0_Counter_K1>"
  Bus Selector2/1 -> P0_ID/1  "<IDP0>"
  Bus Selector2/3 -> P0_dy/1  "<ObjDYP0>"
  Bus Selector2/2 -> P0_dx/1  "<dxP0>"
  Add/1 -> P0_Counter/1
  Constant2/1 -> Add/2
  TrgValidConfirm_inf/1 -> Bus Selector2/1, Bus Selector1/1

== system PubIfDecisionTOS_MDL/TOS_20201112/TOS_2012080320/TOS/P0_Trajectory_V1.0/TrgValidConfirm/TrgValidConfirm/TrgValidConfirm/TrgValidConfirm_Default ==
  Action Port : ActionPort  ActionPortLabel=else
  Constant1 : Constant  Value=0  OutDataTypeStr=single
  Constant2 : Constant  Value=0  OutDataTypeStr=uint32
  Constant3 : Constant  Value=0  OutDataTypeStr=single
  Constant4 : Constant  Value=0  OutDataTypeStr=uint8
  P0_ID : Outport
  P0_Counter : Outport  Port=2
  P0_dx : Outport  Port=3
  P0_dy : Outport  Port=4
  wires:
  Constant1/1 -> P0_dx/1
  Constant4/1 -> P0_ID/1
  Constant3/1 -> P0_dy/1
  Constant2/1 -> P0_Counter/1

== system PubIfDecisionTOS_MDL/TOS_20201112/TOS_2012080320/PIL_1029/BoundaryCalculat/ObjectToCenterLine_dyc/LeftLane/LeftCenterLine_dyc/ObjToCenterLine_dyc_LeftLane/line01_DisJudge ==
  Object_DX : Inport
  line01_dDisStart : Inport  Port=2
  line01_dDisEnd : Inport  Port=3
  Logical Operator : Logic  AllPortsSameDT=off  OutDataTypeStr=boolean
  Relational Operator : RelationalOperator  OutDataTypeStr=boolean  RndMeth=Nearest
  Relational Operator1 : RelationalOperator  Operator=<  OutDataTypeStr=boolean  RndMeth=Nearest
  line01_DisJudge : Outport
  wires:
  Logical Operator/1 -> line01_DisJudge/1
  Relational Operator1/1 -> Logical Operator/2
  Relational Operator/1 -> Logical Operator/1
  Object_DX/1 -> Relational Operator/1, Relational Operator1/1
  line01_dDisStart/1 -> Relational Operator/2
  line01_dDisEnd/1 -> Relational Operator1/2

== system PubIfDecisionTOS_MDL/TOS_20201112/TOS_2012080320/PIL_1029/BoundaryCalculat/ObjectToCenterLine_dyc/LeftLane/LeftCenterLine_dyc/ObjToCenterLine_dyc_LeftLane/line01_dy ==
  Object_DX : Inport
  line01_C0 : Inport  Port=2
  line01_C1 : Inport  Port=3
  line01_C2 : Inport  Port=4
  line01_C3 : Inport  Port=5
  Add : Sum
  Add1 : Sum
  Add3 : Sum
  Constant1 : Constant  Value=3  OutDataTypeStr=single
  Math Function1 : Math  Operator=pow  SignedPower=on  SaturateOnIntegerOverflow=on
  Product : Product
  Product1 : Product
  Product2 : Product
  Square : Math  Operator=square  SignedPower=on  SaturateOnIntegerOverflow=on
  line01_dy : Outport
  wires:
  Add1/1 -> Add/1
  line01_C0/1 -> Add1/1
  Product/1 -> Add/2
  line01_C2/1 -> Product/2
  Square/1 -> Product/1
  Object_DX/1 -> Product1/1, Square/1, Math Function1/1
  Math Function1/1 -> Product2/1
  Product2/1 -> Add3/2
  Product1/1 -> Add1/2
  Constant1/1 -> Math Function1/2
  Add/1 -> Add3/1
  Add3/1 -> line01_dy/1
  line01_C3/1 -> Product2/2
  line01_C1/1 -> Product1/2

== system PubIfDecisionTOS_MDL/TOS_20201112/TOS_2012080320/PIL_1029/BoundaryCalculat/ObjectToCenterLine_dyc/LeftLane/LeftCenterLine_dyc/ObjToCenterLine_dyc_LeftLane/line02_DisJudge ==
  Object_DX : Inport
  line02_dDisStart : Inport  Port=2
  line02_dDisEnd : Inport  Port=3
  Logical Operator : Logic  AllPortsSameDT=off  OutDataTypeStr=boolean
  Relational Operator : RelationalOperator  OutDataTypeStr=boolean  RndMeth=Nearest
  Relational Operator1 : RelationalOperator  Operator=<  OutDataTypeStr=boolean  RndMeth=Nearest
  line02_DisJudge : Outport
  wires:
  line02_dDisEnd/1 -> Relational Operator1/2
  line02_dDisStart/1 -> Relational Operator/2
  Object_DX/1 -> Relational Operator1/1, Relational Operator/1
  Relational Operator/1 -> Logical Operator/1
  Relational Operator1/1 -> Logical Operator/2
  Logical Operator/1 -> line02_DisJudge/1

== system PubIfDecisionTOS_MDL/TOS_20201112/TOS_2012080320/PIL_1029/BoundaryCalculat/ObjectToCenterLine_dyc/LeftLane/LeftCenterLine_dyc/ObjToCenterLine_dyc_LeftLane/line02_dy ==
  Object_DX : Inport
  line02_C0 : Inport  Port=2
  line02_C1 : Inport  Port=3
  line02_C2 : Inport  Port=4
  line02_C3 : Inport  Port=5
  Add : Sum
  Add1 : Sum
  Add3 : Sum
  Constant1 : Constant  Value=3  OutDataTypeStr=single
  Math Function1 : Math  Operator=pow  SignedPower=on  SaturateOnIntegerOverflow=on
  Product : Product
  Product1 : Product
  Product2 : Product
  Square : Math  Operator=square  SignedPower=on  SaturateOnIntegerOverflow=on
  line02_dy : Outport
  wires:
  line02_C1/1 -> Product1/2
  line02_C3/1 -> Product2/2
  Add3/1 -> line02_dy/1
  Add/1 -> Add3/1
  Constant1/1 -> Math Function1/2
  Product1/1 -> Add1/2
  Product2/1 -> Add3/2
  Math Function1/1 -> Product2/1
  Object_DX/1 -> Math Function1/1, Square/1, Product1/1
  Square/1 -> Product/1
  line02_C2/1 -> Product/2
  Product/1 -> Add/2
  line02_C0/1 -> Add1/1
  Add1/1 -> Add/1

== system PubIfDecisionTOS_MDL/TOS_20201112/TOS_2012080320/PIL_1029/BoundaryCalculat/ObjectToCenterLine_dyc/LeftLane/LeftCenterLine_dyc/ObjToCenterLine_dyc_LeftLane/line03_DisJudge ==
  Object_DX : Inport
  line03_dDisStart : Inport  Port=2
  line03_dDisEnd : Inport  Port=3
  Logical Operator : Logic  AllPortsSameDT=off  OutDataTypeStr=boolean
  Relational Operator : RelationalOperator  OutDataTypeStr=boolean  RndMeth=Nearest
  Relational Operator1 : RelationalOperator  Operator=<  OutDataTypeStr=boolean  RndMeth=Nearest
  line03_DisJudge : Outport
  wires:
  Logical Operator/1 -> line03_DisJudge/1
  Relational Operator1/1 -> Logical Operator/2
  Relational Operator/1 -> Logical Operator/1
  Object_DX/1 -> Relational Operator/1, Relational Operator1/1
  line03_dDisStart/1 -> Relational Operator/2
  line03_dDisEnd/1 -> Relational Operator1/2

== system PubIfDecisionTOS_MDL/TOS_20201112/TOS_2012080320/PIL_1029/BoundaryCalculat/ObjectToCenterLine_dyc/LeftLane/LeftCenterLine_dyc/ObjToCenterLine_dyc_LeftLane/line03_dy ==
  Object_DX : Inport
  line03_C0 : Inport  Port=2
  line03_C1 : Inport  Port=3
  line03_C2 : Inport  Port=4
  line03_C3 : Inport  Port=5
  Add : Sum
  Add1 : Sum
  Add3 : Sum
  Constant1 : Constant  Value=3  OutDataTypeStr=single
  Math Function1 : Math  Operator=pow  SignedPower=on  SaturateOnIntegerOverflow=on
  Product : Product
  Product1 : Product
  Product2 : Product
  Square : Math  Operator=square  SignedPower=on  SaturateOnIntegerOverflow=on
  line03_dy : Outport
  wires:
  Add1/1 -> Add/1
  line03_C0/1 -> Add1/1
  Product/1 -> Add/2
  line03_C2/1 -> Product/2
  Square/1 -> Product/1
  Object_DX/1 -> Product1/1, Square/1, Math Function1/1
  Math Function1/1 -> Product2/1
  Product2/1 -> Add3/2
  Product1/1 -> Add1/2
  Constant1/1 -> Math Function1/2
  Add/1 -> Add3/1
  Add3/1 -> line03_dy/1
  line03_C3/1 -> Product2/2
  line03_C1/1 -> Product1/2

== system PubIfDecisionTOS_MDL/TOS_20201112/TOS_2012080320/PIL_1029/BoundaryCalculat/ObjectToCenterLine_dyc/LeftLane/LeftCenterLine_dyc/ObjToCenterLine_dyc_LeftLane/line04_DisJudge ==
  Object_DX : Inport
  line04_dDisStart : Inport  Port=2
  line04_dDisEnd : Inport  Port=3
  Logical Operator : Logic  AllPortsSameDT=off  OutDataTypeStr=boolean
  Relational Operator : RelationalOperator  OutDataTypeStr=boolean  RndMeth=Nearest
  Relational Operator1 : RelationalOperator  Operator=<  OutDataTypeStr=boolean  RndMeth=Nearest
  line04_DisJudge : Outport
  wires:
  line04_dDisEnd/1 -> Relational Operator1/2
  line04_dDisStart/1 -> Relational Operator/2
  Object_DX/1 -> Relational Operator1/1, Relational Operator/1
  Relational Operator/1 -> Logical Operator/1
  Relational Operator1/1 -> Logical Operator/2
  Logical Operator/1 -> line04_DisJudge/1

== system PubIfDecisionTOS_MDL/TOS_20201112/TOS_2012080320/PIL_1029/BoundaryCalculat/ObjectToCenterLine_dyc/LeftLane/LeftCenterLine_dyc/ObjToCenterLine_dyc_LeftLane/line04_dy ==
  Object_DX : Inport
  line04_C0 : Inport  Port=2
  line04_C1 : Inport  Port=3
  line04_C2 : Inport  Port=4
  line04_C3 : Inport  Port=5
  Add : Sum
  Add1 : Sum
  Add3 : Sum
  Constant1 : Constant  Value=3  OutDataTypeStr=single
  Math Function1 : Math  Operator=pow  SignedPower=on  SaturateOnIntegerOverflow=on
  Product : Product
  Product1 : Product
  Product2 : Product
  Square : Math  Operator=square  SignedPower=on  SaturateOnIntegerOverflow=on
  line04_dy : Outport
  wires:
  line04_C1/1 -> Product1/2
  line04_C3/1 -> Product2/2
  Add3/1 -> line04_dy/1
  Add/1 -> Add3/1
  Constant1/1 -> Math Function1/2
  Product1/1 -> Add1/2
  Product2/1 -> Add3/2
  Math Function1/1 -> Product2/1
  Object_DX/1 -> Math Function1/1, Square/1, Product1/1
  Square/1 -> Product/1
  line04_C2/1 -> Product/2
  Product/1 -> Add/2
  line04_C0/1 -> Add1/1
  Add1/1 -> Add/1

== system PubIfDecisionTOS_MDL/TOS_20201112/TOS_2012080320/PIL_1029/BoundaryCalculat/ObjectToCenterLine_dyc/LeftLane/LeftCenterLine_dyc/ObjToCenterLine_dyc_LeftLane/line05_DisJudge ==
  Object_DX : Inport
  line05_dDisStart : Inport  Port=2
  line05_dDisEnd : Inport  Port=3
  Logical Operator : Logic  AllPortsSameDT=off  OutDataTypeStr=boolean
  Relational Operator : RelationalOperator  OutDataTypeStr=boolean  RndMeth=Nearest
  Relational Operator1 : RelationalOperator  Operator=<  OutDataTypeStr=boolean  RndMeth=Nearest
  line05_DisJudge : Outport
  wires:
  Logical Operator/1 -> line05_DisJudge/1
  Relational Operator1/1 -> Logical Operator/2
  Relational Operator/1 -> Logical Operator/1
  Object_DX/1 -> Relational Operator/1, Relational Operator1/1
  line05_dDisStart/1 -> Relational Operator/2
  line05_dDisEnd/1 -> Relational Operator1/2

== system PubIfDecisionTOS_MDL/TOS_20201112/TOS_2012080320/PIL_1029/BoundaryCalculat/ObjectToCenterLine_dyc/LeftLane/LeftCenterLine_dyc/ObjToCenterLine_dyc_LeftLane/line05_dy ==
  Object_DX : Inport
  line05_C0 : Inport  Port=2
  line05_C1 : Inport  Port=3
  line05_C2 : Inport  Port=4
  line05_C3 : Inport  Port=5
  Add : Sum
  Add1 : Sum
  Add3 : Sum
  Constant1 : Constant  Value=3  OutDataTypeStr=single
  Math Function1 : Math  Operator=pow  SignedPower=on  SaturateOnIntegerOverflow=on
  Product : Product
  Product1 : Product
  Product2 : Product
  Square : Math  Operator=square  SignedPower=on  SaturateOnIntegerOverflow=on
  line05_dy : Outport
  wires:
  Add1/1 -> Add/1
  line05_C0/1 -> Add1/1
  Product/1 -> Add/2
  line05_C2/1 -> Product/2
  Square/1 -> Product/1
  Object_DX/1 -> Product1/1, Square/1, Math Function1/1
  Math Function1/1 -> Product2/1
  Product2/1 -> Add3/2
  Product1/1 -> Add1/2
  Constant1/1 -> Math Function1/2
  Add/1 -> Add3/1
  Add3/1 -> line05_dy/1
  line05_C3/1 -> Product2/2
  line05_C1/1 -> Product1/2

== system PubIfDecisionTOS_MDL/TOS_20201112/TOS_2012080320/PIL_1029/BoundaryCalculat/ObjectToCenterLine_dyc/LeftLane/LeftCenterLine_dyc/ObjToCenterLine_dyc_LeftLane/line06_DisJudge ==
  Object_DX : Inport
  line06_dDisStart : Inport  Port=2
  line06_dDisEnd : Inport  Port=3
  Logical Operator : Logic  AllPortsSameDT=off  OutDataTypeStr=boolean
  Relational Operator : RelationalOperator  OutDataTypeStr=boolean  RndMeth=Nearest
  Relational Operator1 : RelationalOperator  Operator=<  OutDataTypeStr=boolean  RndMeth=Nearest
  line06_DisJudge : Outport
  wires:
  line06_dDisEnd/1 -> Relational Operator1/2
  line06_dDisStart/1 -> Relational Operator/2
  Object_DX/1 -> Relational Operator1/1, Relational Operator/1
  Relational Operator/1 -> Logical Operator/1
  Relational Operator1/1 -> Logical Operator/2
  Logical Operator/1 -> line06_DisJudge/1

== system PubIfDecisionTOS_MDL/TOS_20201112/TOS_2012080320/PIL_1029/BoundaryCalculat/ObjectToCenterLine_dyc/LeftLane/LeftCenterLine_dyc/ObjToCenterLine_dyc_LeftLane/line06_dy ==
  Object_DX : Inport
  line06_C0 : Inport  Port=2
  line06_C1 : Inport  Port=3
  line06_C2 : Inport  Port=4
  line6_C3 : Inport  Port=5
  Add : Sum
  Add1 : Sum
  Add3 : Sum
  Constant1 : Constant  Value=3  OutDataTypeStr=single
  Math Function1 : Math  Operator=pow  SignedPower=on  SaturateOnIntegerOverflow=on
  Product : Product
  Product1 : Product
  Product2 : Product
  Square : Math  Operator=square  SignedPower=on  SaturateOnIntegerOverflow=on
  line6_dy : Outport
  wires:
  line06_C1/1 -> Product1/2
  line6_C3/1 -> Product2/2
  Add3/1 -> line6_dy/1
  Add/1 -> Add3/1
  Constant1/1 -> Math Function1/2
  Product1/1 -> Add1/2
  Product2/1 -> Add3/2
  Math Function1/1 -> Product2/1
  Object_DX/1 -> Math Function1/1, Square/1, Product1/1
  Square/1 -> Product/1
  line06_C2/1 -> Product/2
  Product/1 -> Add/2
  line06_C0/1 -> Add1/1
  Add1/1 -> Add/1

== system PubIfDecisionTOS_MDL/TOS_20201112/TOS_2012080320/PIL_1029/BoundaryCalculat/ObjectToCenterLine_dyc/LeftLane/PIL_ObjectToCenterLine_dy_Filt/PIL_ObjectToCenterLine_dy/PP_SignalProcessingDefault ==
  Action Port : ActionPort  ActionPortLabel=if(u1 ~= 0)
  Constant : Constant  Value=0  OutDataTypeStr=uint8
  Constant1 : Constant  Value=255  OutDataTypeStr=single
  Obj_ID : Outport
  ObjectToCenterLine_dy_Filt : Outport  Port=2  OutDataTypeStr=single
  wires:
  Constant1/1 -> ObjectToCenterLine_dy_Filt/1
  Constant/1 -> Obj_ID/1

== system PubIfDecisionTOS_MDL/TOS_20201112/TOS_2012080320/PIL_1029/BoundaryCalculat/ObjectToCenterLine_dyc/LeftLane/PIL_ObjectToCenterLine_dy_Filt/PIL_ObjectToCenterLine_dy/Subsystem ==
  ObjectID_Filt_K1 : Inport
  ObjectToCenterLine_dy_Filt_K1 : Inport  Port=2  OutDataTypeStr=single
  ObjectToCenterLine_dy : Inport  Port=3  OutDataTypeStr=single
  Object_ID : Inport  Port=4  OutDataTypeStr=uint8
  Object_Age : Inport  Port=5
  TOS_OFMObjValid_Flag : Inport  Port=6
  Action Port : ActionPort  ActionPortLabel=else
  Constant1 : Constant  Value=C_TOS_NumberOfEffectiveTargets  OutDataTypeStr=int32
      settings: AttributesFormatString=C_TOS_NumberOfEffectiveTargets = 80
  Constant2 : Constant  Value=0.2  OutDataTypeStr=single
      settings: AttributesFormatString=P_TOS_PIL_ObjectToCenterLine_dy_CutInDeclineLimit = 0.1
  Constant8 : Constant  Value=0.35  OutDataTypeStr=single
      settings: AttributesFormatString=P_TOS_PIL_ObjectToCenterLine_dy_CutInUpperLimit = 0.5
  ObjectToCenterLine_dyFilit : MATLAB Function  TreatAsAtomicUnit=on
  Terminator : Terminator
  Obj_ID : Outport
  ObjectToCenterLine_dy_Filt : Outport  Port=2  OutDataTypeStr=single
  wires:
  TOS_OFMObjValid_Flag/1 -> ObjectToCenterLine_dyFilit/5(TOS_OFMObjValid_Flag)
  Object_Age/1 -> Terminator/1
  ObjectToCenterLine_dy_Filt_K1/1 -> ObjectToCenterLine_dyFilit/2(ObjectToCenterLine_dy_Filt_K1)
  Object_ID/1 -> Obj_ID/1, ObjectToCenterLine_dyFilit/4(Object_ID)
  ObjectID_Filt_K1/1 -> ObjectToCenterLine_dyFilit/1(ObjectID_Filt_K1)
  Constant2/1 -> ObjectToCenterLine_dyFilit/7(P_TOS_PIL_ObjectToCenterLine_dy_CutInDeclineLimit)
  Constant1/1 -> ObjectToCenterLine_dyFilit/8(Iterator_Num)
  ObjectToCenterLine_dy/1 -> ObjectToCenterLine_dyFilit/3(ObjectToCenterLine_dy)
  Constant8/1 -> ObjectToCenterLine_dyFilit/6(P_TOS_PIL_ObjectToCenterLine_dy_CutInUpperLimit)
  ObjectToCenterLine_dyFilit/1(ObjectToCenterLine_dy_Filt) -> ObjectToCenterLine_dy_Filt/1

== system PubIfDecisionTOS_MDL/TOS_20201112/TOS_2012080320/PIL_1029/BoundaryCalculat/ObjectToCenterLine_dyc/RightLane/PIL_ObjectToCenterLine_dy_Filt/PIL_ObjectToCenterLine_dy/PP_SignalProcessingDefault ==
  Action Port : ActionPort  ActionPortLabel=if(u1 ~= 0)
  Constant : Constant  Value=0  OutDataTypeStr=uint8
  Constant1 : Constant  Value=255  OutDataTypeStr=single
  Obj_ID : Outport
  ObjectToCenterLine_dy_Filt : Outport  Port=2  OutDataTypeStr=single
  wires:
  Constant1/1 -> ObjectToCenterLine_dy_Filt/1
  Constant/1 -> Obj_ID/1

== system PubIfDecisionTOS_MDL/TOS_20201112/TOS_2012080320/PIL_1029/BoundaryCalculat/ObjectToCenterLine_dyc/RightLane/PIL_ObjectToCenterLine_dy_Filt/PIL_ObjectToCenterLine_dy/Subsystem ==
  ObjectID_Filt_K1 : Inport
  ObjectToCenterLine_dy_Filt_K1 : Inport  Port=2  OutDataTypeStr=single
  ObjectToCenterLine_dy : Inport  Port=3  OutDataTypeStr=single
  Object_ID : Inport  Port=4  OutDataTypeStr=uint8
  Object_Age : Inport  Port=5
  TOS_OFMObjValid_Flag : Inport  Port=6
  Action Port : ActionPort  ActionPortLabel=else
  Constant1 : Constant  Value=C_TOS_NumberOfEffectiveTargets  OutDataTypeStr=int32
      settings: AttributesFormatString=C_TOS_NumberOfEffectiveTargets = 80
  Constant2 : Constant  Value=0.2  OutDataTypeStr=single
      settings: AttributesFormatString=P_TOS_PIL_ObjectToCenterLine_dy_CutInDeclineLimit = 0.1
  Constant8 : Constant  Value=0.35  OutDataTypeStr=single
      settings: AttributesFormatString=P_TOS_PIL_ObjectToCenterLine_dy_CutInUpperLimit = 0.5
  ObjectToCenterLine_dyFilit : MATLAB Function  TreatAsAtomicUnit=on
  Terminator : Terminator
  Obj_ID : Outport
  ObjectToCenterLine_dy_Filt : Outport  Port=2  OutDataTypeStr=single
  wires:
  TOS_OFMObjValid_Flag/1 -> ObjectToCenterLine_dyFilit/5(TOS_OFMObjValid_Flag)
  Object_Age/1 -> Terminator/1
  ObjectToCenterLine_dy_Filt_K1/1 -> ObjectToCenterLine_dyFilit/2(ObjectToCenterLine_dy_Filt_K1)
  Object_ID/1 -> Obj_ID/1, ObjectToCenterLine_dyFilit/4(Object_ID)
  ObjectID_Filt_K1/1 -> ObjectToCenterLine_dyFilit/1(ObjectID_Filt_K1)
  Constant2/1 -> ObjectToCenterLine_dyFilit/7(P_TOS_PIL_ObjectToCenterLine_dy_CutInDeclineLimit)
  Constant1/1 -> ObjectToCenterLine_dyFilit/8(Iterator_Num)
  ObjectToCenterLine_dy/1 -> ObjectToCenterLine_dyFilit/3(ObjectToCenterLine_dy)
  Constant8/1 -> ObjectToCenterLine_dyFilit/6(P_TOS_PIL_ObjectToCenterLine_dy_CutInUpperLimit)
  ObjectToCenterLine_dyFilit/1(ObjectToCenterLine_dy_Filt) -> ObjectToCenterLine_dy_Filt/1

== system PubIfDecisionTOS_MDL/TOS_20201112/TOS_2012080320/PIL_1029/BoundaryCalculat/ObjectToCenterLine_dyc/RightLane/RightCenterLine_dyc/ObjToCenterLine_dyc_RightLane/line01_DisJudge ==
  Object_DX : Inport
  line01_dDisStart : Inport  Port=2
  line01_dDisEnd : Inport  Port=3
  Logical Operator : Logic  AllPortsSameDT=off  OutDataTypeStr=boolean
  Relational Operator : RelationalOperator  OutDataTypeStr=boolean  RndMeth=Nearest
  Relational Operator1 : RelationalOperator  Operator=<  OutDataTypeStr=boolean  RndMeth=Nearest
  line01_DisJudge : Outport
  wires:
  line01_dDisEnd/1 -> Relational Operator1/2
  line01_dDisStart/1 -> Relational Operator/2
  Object_DX/1 -> Relational Operator1/1, Relational Operator/1
  Relational Operator/1 -> Logical Operator/1
  Relational Operator1/1 -> Logical Operator/2
  Logical Operator/1 -> line01_DisJudge/1
